simulink model "netra_district"  (R2026a)
settings: Solver=FixedStepDiscrete  StartTime=0  StopTime=250  FixedStep=1
settings Model: Creator=kanha  LastModifiedBy=kanha

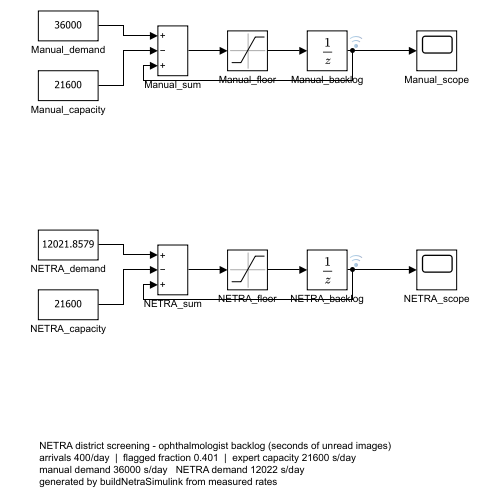
[thumbnail: Simulink's stored preview of the top-level diagram]
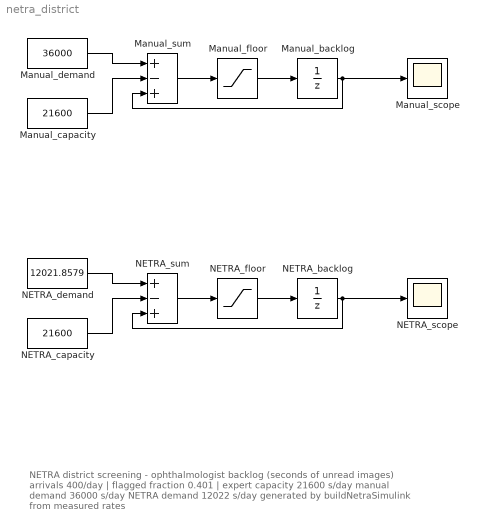
== system netra_district ==
  note: NETRA district screening - ophthalmologist backlog (seconds of unread images)
      | arrivals 400/day  |  flagged fraction 0.401  |  expert capacity 21600 s/day
      | manual demand 36000 s/day   NETRA demand 12022 s/day
      | generated by buildNetraSimulink from measured rates
  Manual_backlog : UnitDelay  SampleTime=-1
  Manual_capacity : Constant  Value=21600
  Manual_demand : Constant  Value=36000
  Manual_floor : Saturate  UpperLimit=inf  LowerLimit=0
  Manual_scope : Scope
  Manual_sum : Sum  Inputs=+-+
  NETRA_backlog : UnitDelay  SampleTime=-1
  NETRA_capacity : Constant  Value=21600
  NETRA_demand : Constant  Value=12021.8579
  NETRA_floor : Saturate  UpperLimit=inf  LowerLimit=0
  NETRA_scope : Scope
  NETRA_sum : Sum  Inputs=+-+
  wires:
  Manual_demand/1 -> Manual_sum/1
  Manual_capacity/1 -> Manual_sum/2
  Manual_sum/1 -> Manual_floor/1
  Manual_floor/1 -> Manual_backlog/1
  Manual_backlog/1 -> Manual_scope/1, Manual_sum/3
  NETRA_demand/1 -> NETRA_sum/1
  NETRA_capacity/1 -> NETRA_sum/2
  NETRA_sum/1 -> NETRA_floor/1
  NETRA_floor/1 -> NETRA_backlog/1
  NETRA_backlog/1 -> NETRA_scope/1, NETRA_sum/3
